simulink model "model_expanded_breach"  (R2017a)
settings: Solver=FixedStepAuto  StartTime=0.0  StopTime=30.0  RelTol=1e-3  EnableMultiTasking=on
model workspace: external: MAT-File model_expanded_params.mat (data not in the file)
undefined symbols (not defined in the file or in its folder): a, b, g, Kf, Km, m
settings Model: Creator=Felipe Vargas  LastModifiedBy=nikhil
settings DataIOCC: LimitDataPoints=on  SaveFormat=Array
settings OptimizationCC: LifeSpan=inf
settings DebuggingCC: SFUnexpectedBacktrackingDiag=warning  SFNoUnconditionalDefaultTransitionDiag=warning  SFExecutionAtInitializationDiag=none
settings HardwareCC: ProdBitPerPointer=32  ProdBitPerSizeT=32  ProdBitPerPtrDiffT=32  ProdLargestAtomicFloat=None  ProdIntDivRoundTo=Undefined  ProdEndianess=Unspecified  ProdWordSize=32  ProdHWDeviceType=32-bit Generic
settings ModelReferenceCC: PropagateSignalLabelsOutOfModel=off
settings GRTTargetCC: TargetLangStandard=C89/C90 (ANSI)  GeneratePreprocessorConditionals=Disable all
settings ConfigComp: CovMetricSettings=dw  CovHtmlReporting=on  CovSaveCumulativeToWorkspaceVar=on  CovSaveSingleToWorkspaceVar=on  CovExternalEMLEnable=off

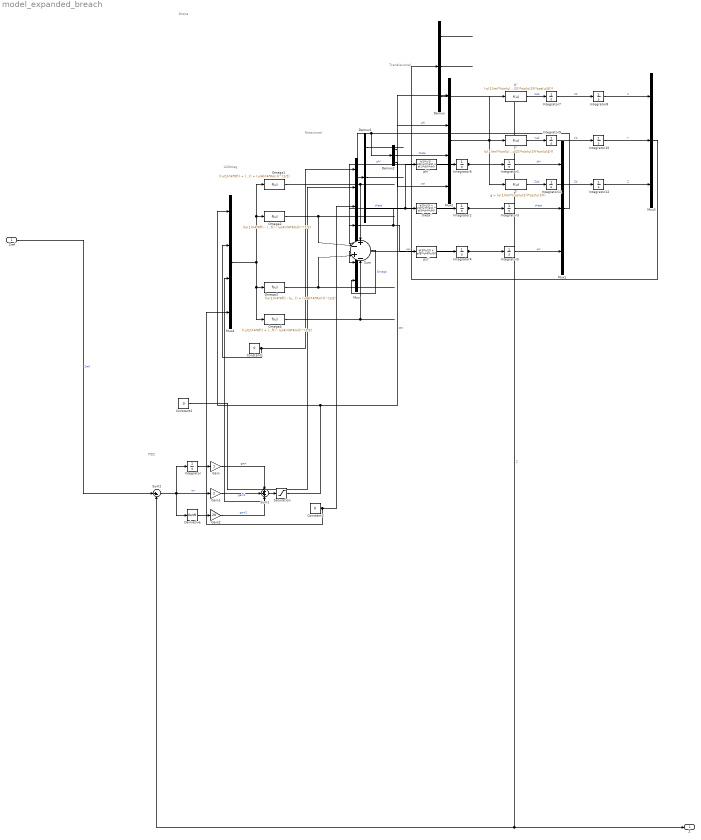
== system model_expanded_breach ==
  note: U2Omeg
  note: Translacional
  note: Rotacional
  note: PIDZ
  note: Drone
  Zref : Inport
  Constant1 : Constant  Value=0
  Constant2 : Constant  Value=0
  Constant3 : Constant  Value=0
  Demux : Demux  Outputs=3
  Demux1 : Demux  Outputs=3
  Demux2 : Demux  Outputs=3
  Derivative : Derivative
  Gain : Gain
  Gain1 : Gain  Gain=2
  Gain2 : Gain  Gain=20
  Integrator{,1..12} (13 alike) : Integrator
  Mux : Mux  Inputs=7
  Mux1 : Mux  Inputs=3
  Mux2 : Mux
  Mux3 : Mux  Inputs=3
  Mux4 : Mux
  Omega1 : Fcn  Expr=((u(1)/(4*Kf)) + (u(3)/(2*Kf)) + (u(4)/(4*Km)))^(1/2)
  Omega2 : Fcn  Expr=((u(1)/(4*Kf)) - (u(2)/(2*Kf)) - (u(4)/(4*Km)))^(1/2)
  Omega3 : Fcn  Expr=((u(1)/(4*Kf)) - (u(3)/(2*Kf)) + (u(4)/(4*Km)))^(1/2)
  Omega4 : Fcn  Expr=((u(1)/(4*Kf)) + (u(2)/(2*Kf)) - (u(4)/(4*Km)))^(1/2)
  Saturation : Saturate  UpperLimit=15  LowerLimit=-15
  Sum : Sum  Inputs=+-+-
  Sum1 : Sum  Inputs=+++
  Sum2 : Sum  Inputs=|+-
  X'' : Fcn  Expr=(-u(1)/m)*(sin(u(2))*sin(u(4)) + cos(u(2))*sin(u(3))*cos(u(4)))
  Y'' : Fcn  Expr=(u(1)/m)*(sin(u(2))*cos(u(4)) - cos(u(2))*sin(u(3))*sin(u(4)))
  Z'' : Fcn  Expr=g + (u(1)/m)*(cos(u(2))*cos(u(3)))
  phi'' : Fcn  Expr=b(1)*u(1) - u(5)*u(7)*a(2) + a(1)*u(5)*u(6)
  psi'' : Fcn  Expr=b(3)*u(3) + a(5)*u(4)*u(5)
  theta'' : Fcn  Expr=b(2)*u(2) + u(4)*u(7)*a(4) + a(3)*u(4)*u(6)
  Z : Outport
  wires:
  Demux/3 -> Z/1, Sum2/2  "Z"
  Zref/1 -> Sum2/1  "Zref"
  Demux/2 -> ?
  Demux/1 -> ?
  Mux3/1 -> Demux/1
  Demux1/3 -> ?
  Demux1/2 -> ?
  Demux1/1 -> ?
  Saturation/1 -> Mux2/1, Mux4/1  "sat"
  Gain/1 -> Sum1/1  "gain"
  Sum1/1 -> Saturation/1
  Gain1/1 -> Sum1/2  "gain1"
  Derivative/1 -> Gain2/1
  Sum2/1 -> Derivative/1, Gain1/1, Integrator/1  "err"
  Gain2/1 -> Sum1/3  "gain2"
  Integrator/1 -> Gain/1
  Integrator5/1 -> Mux1/3  "psi"
  Integrator3/1 -> Mux1/2  "theta"
  Integrator1/1 -> Mux1/1  "phi"
  Integrator4/1 -> Integrator5/1, Mux/6  "psi'"
  psi''/1 -> Integrator4/1
  Integrator2/1 -> Integrator3/1, Mux/5  "theta'"
  theta''/1 -> Integrator2/1
  Mux/1 -> psi''/1, theta''/1, phi''/1
  Integrator6/1 -> Integrator1/1, Mux/4  "phi'"
  phi''/1 -> Integrator6/1
  Integrator12/1 -> Mux3/3  "Z"
  Integrator11/1 -> Integrator12/1  "Zd"
  Z''/1 -> Integrator11/1  "Zdd"
  Integrator10/1 -> Mux3/2  "Y"
  Integrator9/1 -> Integrator10/1  "Yd"
  Y''/1 -> Integrator9/1  "Ydd"
  Demux2/3 -> Mux2/4  "psi"
  Demux2/2 -> Mux2/3  "theta"
  Demux2/1 -> Mux2/2  "phi"
  Mux2/1 -> Z''/1, Y''/1, X''/1
  Mux1/1 -> Demux1/1, Demux2/1
  Integrator8/1 -> Mux3/1  "X"
  Integrator7/1 -> Integrator8/1  "Xd"
  X''/1 -> Integrator7/1  "Xdd"
  Sum/1 -> Mux/7  "Omega"
  Constant1/1 -> Mux4/2, Mux/1
  Constant2/1 -> Mux4/3, Mux/2
  Constant3/1 -> Mux4/4, Mux/3
  Omega4/1 -> Sum/4
  Mux4/1 -> Omega2/1, Omega1/1, Omega4/1, Omega3/1
  Omega3/1 -> Sum/3
  Omega1/1 -> Sum/1
  Omega2/1 -> Sum/2
